simulink model "sensor_model"  (R2021a)
settings: Solver=FixedStepDiscrete  StartTime=0  StopTime=10.0  FixedStep=T_sample_control  RelTol=1e-3  EnableMultiTasking=on
model workspace (MAT data in the model file):
  CG = [0 0 0]
  g = [0 0 -9.81]
  t_sensor = 0.001
undefined symbols (not defined in the file or in its folder): DiscIntNeverNeededParam
libraries: rotations_lib x6, mspfiltlib x2, mspsensorlib x2, robotcorelib x2, aerolibcommonsys x1
settings Model: DataDictionary=pid.sldd  EnableAccessToBaseWorkspace=off  ModifiedByFormat=The MathWorks Inc.  Creator=The MathWorks, Inc.  LastModifiedBy=The MathWorks Inc.
settings SolverCC: ZeroCrossControl=DisableAll  AlgebraicLoopSolver=TrustRegion
settings DataIOCC: SaveFormat=StructureWithTime  SaveOutput=off  SaveTime=off  ReturnWorkspaceOutputs=off
settings OptimizationCC: BlockReduction=off  DefaultParameterBehavior=Inlined  InlineInvariantSignals=on  BufferReuse=off  PassReuseOutputArgsAs=Individual arguments  ExpressionDepthLimit=2147483647  ZeroExternalMemoryAtStartup=off  ZeroInternalMemoryAtStartup=off  EfficientFloat2IntCast=on  LifeSpan=1  EfficientTunableParamExpr=on
settings DebuggingCC: AlgebraicLoopMsg=none  FcnCallInpInsideContextMsg=warning  UnconnectedInputMsg=none  UnconnectedOutputMsg=none  UnconnectedLineMsg=none  UniqueDataStoreMsg=error  AssertControl=DisableAll  AllowSymbolicDim=off  StateNameClashWarn=warning  StrictBusMsg=ErrorOnBusTreatedAsVector  SFUnexpectedBacktrackingDiag=warning  SFNoUnconditionalDefaultTransitionDiag=warning  SFExecutionAtInitializationDiag=none  SFMachineParentedDataDiag=warning  ArithmeticOperatorsInVariantConditions=warning
settings HardwareCC: ProdBitPerPointer=32  ProdBitPerSizeT=32  ProdBitPerPtrDiffT=32  ProdLargestAtomicFloat=None  ProdIntDivRoundTo=Undefined  ProdEndianess=Unspecified  ProdWordSize=32  ProdHWDeviceType=32-bit Generic
settings ModelReferenceCC: PropagateSignalLabelsOutOfModel=off
settings SFSimCC: SimUseLocalCustomCode=off  CustomCodeUndefinedFunction=UseInterfaceOnly
settings RTWCC: SystemTargetFile=ert.tlc  TemplateMakefile=ert_default_tmf  GenerateReport=on  RTWUseLocalCustomCode=off  IncludeHyperlinkInReport=on  GenerateTraceInfo=on  GenerateTraceReport=on  GenerateTraceReportSl=on  GenerateTraceReportSf=on  GenerateTraceReportEml=on  GenerateCodeMetricsReport=on
settings CodeAppCC: IgnoreCustomStorageClasses=off  IgnoreTestpoints=on  CustomSymbolStrType=$N$R$M  StateflowObjectComments=on  InternalIdentifier=Classic
settings ERTTargetCC: MultiwordLength=2048  GenerateSampleERTMain=on  CombineOutputUpdateFcns=off  SupportNonFinite=off  ParenthesesLevel=Maximum  InlinedParameterPlacement=NonHierarchical  ERTCustomFileTemplate=example_file_process.tlc  ConvertIfToSwitch=off  SuppressUnreachableDefaultCases=off
settings ConfigComp: CovMetricSettings=dw  CovSaveCumulativeToWorkspaceVar=on  CovSaveSingleToWorkspaceVar=on  CovExternalEMLEnable=off  CovSFcnEnable=off

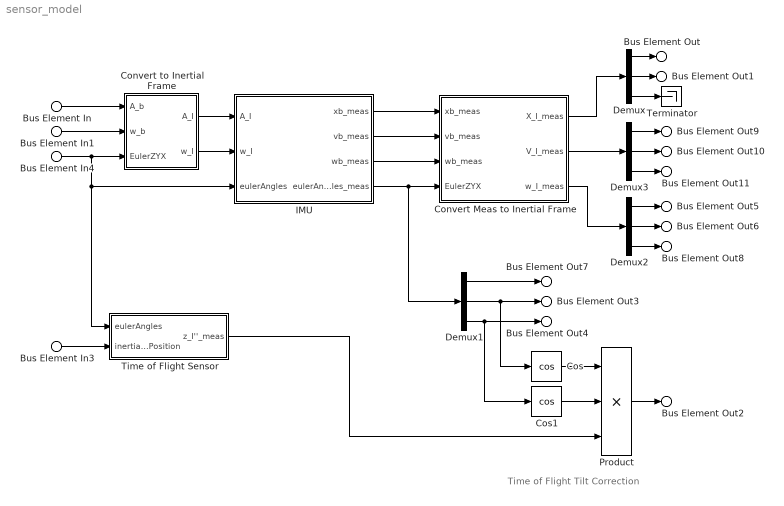
== system sensor_model ==
  note: Time of Flight Tilt Correction
  Bus Element In : Inport  PortName=6DOF  Element=body.acceleration
  Bus Element In1 : Inport  PortName=6DOF  Element=body.angularRate
  Bus Element In4 : Inport  PortName=6DOF  Element=body.angles
  Bus Element In3 : Inport  PortName=6DOF  Element=inertial.position
  Convert Meas to Inertial Frame : Subsystem
  Convert to Inertial Frame : Subsystem
  Cos : Trigonometry  Operator=cos
  Cos1 : Trigonometry  Operator=cos
  Demux{,1..3} (4 alike) : Demux  Outputs=3
  IMU : Subsystem  Description=Model approximating the SparkFun 9DoF IMU (ICM-20948) which will be used to determine the XY position and velocity and the attitude and angular rates of the flyer. The model uses the IMU and Attitude and Heading Reference System (AHRS) Simulink blocks to simulate our sensor.
  Product : Product  Inputs=3
  Terminator : Terminator
  Time of Flight Sensor : Subsystem  Description=A simulation model of the VL53L1X Time of Flight (ToF) sensor which determines the distance of the MFWF to the ground.
  Bus Element Out : Outport  PortName=sensor_meas  Element=x
  Bus Element Out1 : Outport  PortName=sensor_meas  Element=y
  Bus Element Out7 : Outport  PortName=sensor_meas  Element=psi
  Bus Element Out3 : Outport  PortName=sensor_meas  Element=theta
  Bus Element Out4 : Outport  PortName=sensor_meas  Element=phi
  Bus Element Out5 : Outport  PortName=sensor_meas  Element=p
  Bus Element Out6 : Outport  PortName=sensor_meas  Element=q
  Bus Element Out8 : Outport  PortName=sensor_meas  Element=r
  Bus Element Out9 : Outport  PortName=sensor_meas  Element=Vx
  Bus Element Out10 : Outport  PortName=sensor_meas  Element=Vy
  Bus Element Out11 : Outport  PortName=sensor_meas  Element=Vz
  Bus Element Out2 : Outport  PortName=sensor_meas  Element=z
  wires:
  Demux/1 -> Bus Element Out/1
  Demux3/3 -> Bus Element Out11/1
  Demux/3 -> Terminator/1
  Demux2/2 -> Bus Element Out6/1
  Demux2/1 -> Bus Element Out5/1
  Demux1/2 -> Bus Element Out3/1, Cos/1
  Demux3/1 -> Bus Element Out9/1
  IMU/4(eulerAngles_meas) -> Demux1/1, Convert Meas to Inertial Frame/4(EulerZYX)
  Demux3/2 -> Bus Element Out10/1
  Demux/2 -> Bus Element Out1/1
  Demux2/3 -> Bus Element Out8/1
  Bus Element In3/1 -> Time of Flight Sensor/2(inertialPosition)
  Bus Element In/1 -> Convert to Inertial Frame/1(A_b)
  Bus Element In1/1 -> Convert to Inertial Frame/2(w_b)
  Convert to Inertial Frame/2(w_I) -> IMU/2(w_I)
  IMU/1(xb_meas) -> Convert Meas to Inertial Frame/1(xb_meas)
  IMU/2(vb_meas) -> Convert Meas to Inertial Frame/2(vb_meas)
  IMU/3(wb_meas) -> Convert Meas to Inertial Frame/3(wb_meas)
  Convert Meas to Inertial Frame/1(X_I_meas) -> Demux/1
  Convert Meas to Inertial Frame/3(w_I_meas) -> Demux2/1
  Cos/1 -> Product/1
  Time of Flight Sensor/1(z_I''_meas) -> Product/3
  Cos1/1 -> Product/2
  Product/1 -> Bus Element Out2/1
  Convert to Inertial Frame/1(A_I) -> IMU/1(A_I)
  Bus Element In4/1 -> Time of Flight Sensor/1(eulerAngles), IMU/3(eulerAngles), Convert to Inertial Frame/3(EulerZYX)
  Convert Meas to Inertial Frame/2(V_I_meas) -> Demux3/1
  Demux1/1 -> Bus Element Out7/1
  Demux1/3 -> Cos1/1, Bus Element Out4/1

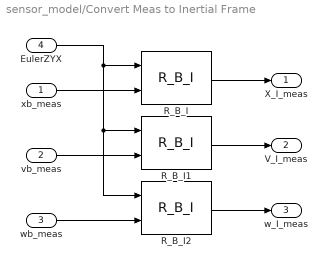
== system sensor_model/Convert Meas to Inertial Frame ==
  xb_meas : Inport
  vb_meas : Inport  Port=2
  wb_meas : Inport  Port=3
  EulerZYX : Inport  Port=4
  R_B_I : rotations_lib/R_B_I  SystemSampleTime=-1  VariantActivationTime=update diagram  Latency=0  AutoFrameSizeCalculation=off
  R_B_I1 : rotations_lib/R_B_I  SystemSampleTime=-1  VariantActivationTime=update diagram  Latency=0  AutoFrameSizeCalculation=off
  R_B_I2 : rotations_lib/R_B_I  SystemSampleTime=-1  VariantActivationTime=update diagram  Latency=0  AutoFrameSizeCalculation=off
  X_I_meas : Outport
  V_I_meas : Outport  Port=2
  w_I_meas : Outport  Port=3
  wires:
  EulerZYX/1 -> R_B_I2/1, R_B_I1/1, R_B_I/1
  xb_meas/1 -> R_B_I/2
  R_B_I/1 -> X_I_meas/1
  vb_meas/1 -> R_B_I1/2
  R_B_I1/1 -> V_I_meas/1
  R_B_I2/1 -> w_I_meas/1
  wb_meas/1 -> R_B_I2/2

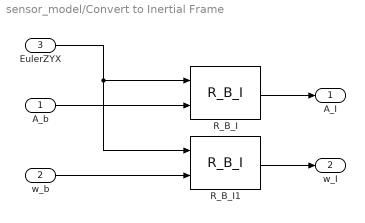
== system sensor_model/Convert to Inertial Frame ==
  A_b : Inport
  w_b : Inport  Port=2
  EulerZYX : Inport  Port=3
  R_B_I : rotations_lib/R_B_I  SystemSampleTime=-1  VariantActivationTime=update diagram  Latency=0  AutoFrameSizeCalculation=off
  R_B_I1 : rotations_lib/R_B_I  SystemSampleTime=-1  VariantActivationTime=update diagram  Latency=0  AutoFrameSizeCalculation=off
  A_I : Outport
  w_I : Outport  Port=2
  wires:
  EulerZYX/1 -> R_B_I1/1, R_B_I/1
  R_B_I/1 -> A_I/1
  A_b/1 -> R_B_I/2
  R_B_I1/1 -> w_I/1
  w_b/1 -> R_B_I1/2

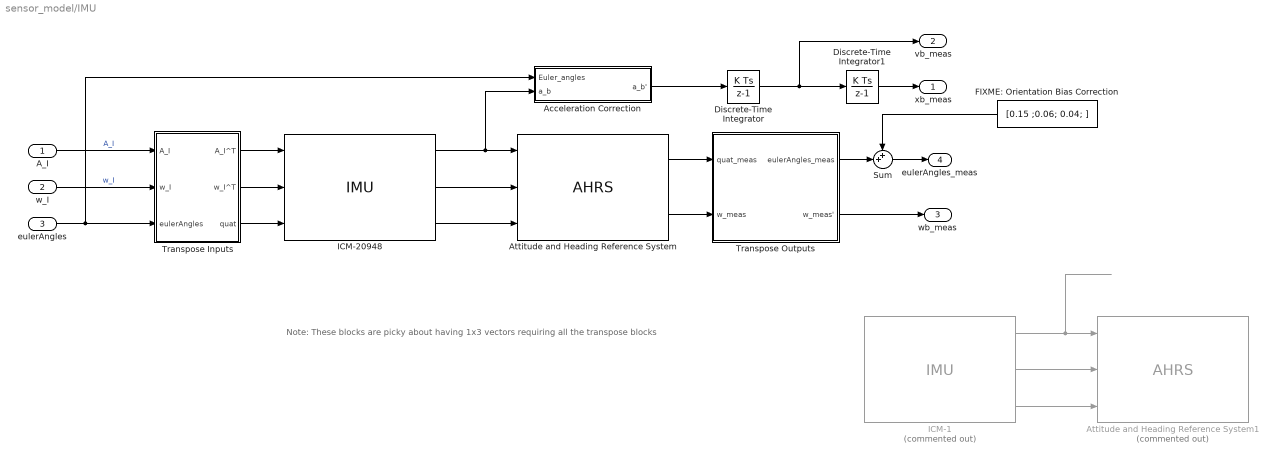
== system sensor_model/IMU ==
  note: Note: These blocks are picky about having 1x3 vectors requiring all the transpose blocks
  A_I : Inport
  w_I : Inport  Port=2
  eulerAngles : Inport  Port=3
  Acceleration Correction : Subsystem
  Attitude and Heading Reference System : mspfiltlib/AHRS  DispRefFrame=ENU  DecimationFactor=1  InitialProcessNoise=ahrsfilter.defaultProcessNoise  OrientationFormat=quaternion  SimulateUsing=Interpreted execution  AccelerometerNoise=0.0050625  GyroscopeNoise=6.84e-5  MagnetometerNoise=0.1e-15  GyroscopeDriftNoise=0.0872  LinearAccelerationNoise=0.55  MagneticDisturbanceNoise=0.3  LinearAccelerationDecayFactor=0.35  MagneticDisturbanceDecayFactor=0.3  ExpectedMagneticFieldStrength=50
      settings: SourceProductBaseCode=TF,NV
  Attitude and Heading Reference System1 : mspfiltlib/AHRS  Commented=on  DispRefFrame=ENU  DecimationFactor=1  InitialProcessNoise=ahrsfilter.defaultProcessNoise  OrientationFormat=quaternion  SimulateUsing=Interpreted execution  AccelerometerNoise=0.0050625  GyroscopeNoise=6.84e-5  MagnetometerNoise=0.1e-15  GyroscopeDriftNoise=0.0872  LinearAccelerationNoise=0.3  MagneticDisturbanceNoise=0.3  LinearAccelerationDecayFactor=0.3  MagneticDisturbanceDecayFactor=0.5  ExpectedMagneticFieldStrength=50
      settings: SourceProductBaseCode=TF,NV
  Discrete-Time Integrator : DiscreteIntegrator  SampleTime=-1  ICPrevOutput=DiscIntNeverNeededParam  ICPrevScaledInput=DiscIntNeverNeededParam
  Discrete-Time Integrator1 : DiscreteIntegrator  SampleTime=-1  ICPrevOutput=DiscIntNeverNeededParam  ICPrevScaledInput=DiscIntNeverNeededParam
  FIXME: Orientation Bias Correction : Constant  Value=[0.15 ;0.06; 0.04; ]
  ICM-1 : mspsensorlib/IMU  Commented=on  DispRefFrame=ENU  Temperature=25  MagneticFieldNED=[ 27.5550, -2.4169, -16.0849 ]  MagneticFieldENU=[ -2.4169, 27.5550, 16.0849 ]  SeedDouble=19  SimulateUsing=Interpreted execution  AccelParamsMeasurementRange=4*9.81  AccelParamsResolution=9.81/8192  AccelParamsConstantBias=[ 0, 0, 0 ]  AccelParamsAxesMisalignment=[ 0, 0, 0 ]  AccelParamsNoiseDensity=[ 230, 230, 230 ] * 9.81e-6  AccelParamsBiasInstability=[ 50, 50, 50] * 9.81e-3  AccelParamsRandomWalk=[ 230, 230, 230 ] * 9.81e-6  AccelParamsTemperatureBias=[ 0.8, 0.8, 0.8 ] * 9.81e-3  AccelParamsTemperatureScaleFactor=[0.026 0.026 0.026]  GyroParamsMeasurementRange=deg2rad(250)  GyroParamsResolution=1/deg2rad(131)  GyroParamsConstantBias=[ 0, 0, 0 ]  GyroParamsAxesMisalignment=[ 0, 0, 0 ]  GyroParamsAccelerationBias=[ 0, 0, 0 ]  GyroParamsNoiseDensity=[ deg2rad(0.015), deg2rad(0.015), deg2rad(0.015) ]  GyroParamsBiasInstability=[ deg2rad(5) , deg2rad(5), deg2rad(5) ]  GyroParamsRandomWalk=[ deg2rad(0.015), deg2rad(0.015), deg2rad(0.015) ]  GyroParamsTemperatureBias=[ deg2rad(0.05), deg2rad(0.05), deg2rad(0.05) ]  GyroParamsTemperatureScaleFactor=[ 3, 3, 3 ]  MagParamsMeasurementRange=4900  MagParamsResolution=0.15  MagParamsConstantBias=[ 0, 0, 0 ]  MagParamsAxesMisalignment=[ 0, 0, 0 ]  MagParamsNoiseDensity=[ 0, 0, 0 ]  MagParamsBiasInstability=[ 0, 0, 0 ]  MagParamsRandomWalk=[ 0, 0, 0 ]  MagParamsTemperatureBias=[ 0, 0, 0 ]  MagParamsTemperatureScaleFactor=[ 0, 0, 0 ]
      settings: SourceProductBaseCode=TF,NV
  ICM-20948 : mspsensorlib/IMU  DispRefFrame=ENU  Temperature=25  MagneticFieldNED=[ 27.5550, -2.4169, -16.0849 ]  MagneticFieldENU=[ -2.4169, 27.5550, 16.0849 ]  SeedDouble=19  SimulateUsing=Interpreted execution  AccelParamsMeasurementRange=4*9.81  AccelParamsResolution=9.81/8192  AccelParamsConstantBias=[ 0, 0, 0 ]  AccelParamsAxesMisalignment=[ 0, 0, 0 ]  AccelParamsNoiseDensity=[ 0, 0, 0 ] * 9.81e-6  AccelParamsBiasInstability=[ 0, 0, 0 ]* 9.81e-3  AccelParamsRandomWalk=[ 0, 0, 0 ]* 9.81e-6  AccelParamsTemperatureBias=[ 0, 0, 0 ]* 9.81e-3  AccelParamsTemperatureScaleFactor=[0.026 0.026 0.026]  GyroParamsMeasurementRange=deg2rad(250)  GyroParamsResolution=1/deg2rad(131)  GyroParamsConstantBias=[ 0, 0, 0 ]  GyroParamsAxesMisalignment=[ 0, 0, 0 ]  GyroParamsAccelerationBias=[ 0, 0, 0 ]  GyroParamsNoiseDensity=[ 0, 0, 0 ]  GyroParamsBiasInstability=[ 0, 0, 0 ]  GyroParamsRandomWalk=[ 0, 0, 0 ]  GyroParamsTemperatureBias=[ 0, 0, 0 ]  GyroParamsTemperatureScaleFactor=[ 0, 0, 0 ]  MagParamsMeasurementRange=4900  MagParamsResolution=0.15  MagParamsConstantBias=[ 0, 0, 0 ]  MagParamsAxesMisalignment=[ 0, 0, 0 ]  MagParamsNoiseDensity=[ 0, 0, 0 ]  MagParamsBiasInstability=[ 0, 0, 0 ]  MagParamsRandomWalk=[ 0, 0, 0 ]  MagParamsTemperatureBias=[ 0, 0, 0 ]  MagParamsTemperatureScaleFactor=[ 0, 0, 0 ]
      settings: SourceProductBaseCode=TF,NV
  Sum : Sum  Inputs=++|
  Transpose Inputs : Subsystem
  Transpose Outputs : Subsystem
  xb_meas : Outport
  vb_meas : Outport  Port=2
  wb_meas : Outport  Port=3
  eulerAngles_meas : Outport  Port=4
  wires:
  ICM-20948/1 -> Acceleration Correction/2(a_b), Attitude and Heading Reference System/1
  ICM-20948/2 -> Attitude and Heading Reference System/2
  ICM-20948/3 -> Attitude and Heading Reference System/3
  Discrete-Time Integrator1/1 -> xb_meas/1
  Discrete-Time Integrator/1 -> Discrete-Time Integrator1/1, vb_meas/1
  eulerAngles/1 -> Acceleration Correction/1(Euler_angles), Transpose Inputs/3(eulerAngles)
  A_I/1 -> Transpose Inputs/1(A_I)  "A_I"
  w_I/1 -> Transpose Inputs/2(w_I)  "w_I"
  Transpose Inputs/1(A_I^T) -> ICM-20948/1
  Transpose Inputs/2(w_I^T) -> ICM-20948/2
  Transpose Inputs/3(quat) -> ICM-20948/3
  Attitude and Heading Reference System/1 -> Transpose Outputs/1(quat_meas)
  Attitude and Heading Reference System/2 -> Transpose Outputs/2(w_meas)
  Transpose Outputs/1(eulerAngles_meas) -> Sum/2
  Transpose Outputs/2(w_meas') -> wb_meas/1
  FIXME: Orientation Bias Correction/1 -> Sum/1
  Acceleration Correction/1(a_b') -> Discrete-Time Integrator/1
  Sum/1 -> eulerAngles_meas/1
  ICM-1/3 -> Attitude and Heading Reference System1/3
  ICM-1/2 -> Attitude and Heading Reference System1/2
  ICM-1/1 -> Attitude and Heading Reference System1/1

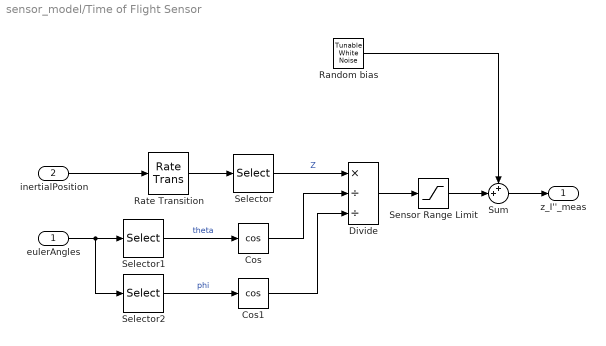
== system sensor_model/Time of Flight Sensor ==
  eulerAngles : Inport
  inertialPosition : Inport  Port=2
  Cos : Trigonometry  Operator=cos
  Cos1 : Trigonometry  Operator=cos
  Divide : Product  Inputs=*//
  Random bias : aerolibcommonsys/Tunable White Noise  pwr=0.0000001  Ts=t_sensor  seed=1337
      settings: SourceProductBaseCode=AE
  Rate Transition : RateTransition  OutPortSampleTime=t_sensor
  Selector : Selector  InputPortWidth=3  IndexOptions=Index vector (dialog)  Indices=[3]  OutputSizes=1
  Selector1 : Selector  InputPortWidth=3  IndexOptions=Index vector (dialog)  Indices=[2]  OutputSizes=1
  Selector2 : Selector  InputPortWidth=3  IndexOptions=Index vector (dialog)  Indices=[3]  OutputSizes=1
  Sensor Range Limit : Saturate  UpperLimit=2.2  LowerLimit=0
  Sum : Sum  Inputs=++|
  z_I''_meas : Outport
  wires:
  inertialPosition/1 -> Rate Transition/1
  Sum/1 -> z_I''_meas/1
  Selector/1 -> Divide/1  "Z"
  Random bias/1 -> Sum/1
  Rate Transition/1 -> Selector/1
  eulerAngles/1 -> Selector2/1, Selector1/1
  Selector1/1 -> Cos/1  "theta"
  Cos/1 -> Divide/2
  Divide/1 -> Sensor Range Limit/1
  Sensor Range Limit/1 -> Sum/2
  Selector2/1 -> Cos1/1  "phi"
  Cos1/1 -> Divide/3

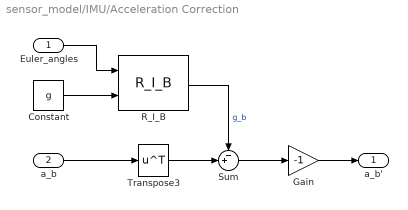
== system sensor_model/IMU/Acceleration Correction ==
  Euler_angles : Inport
  a_b : Inport  Port=2
  Constant : Constant  Value=g
  Gain : Gain  Gain=-1
  R_I_B : rotations_lib/R_I_B  SystemSampleTime=-1  VariantActivationTime=update diagram  Latency=0  AutoFrameSizeCalculation=off
  Sum : Sum  Inputs=-+|
  Transpose3 : Math  Operator=transpose  SaturateOnIntegerOverflow=on
  a_b' : Outport
  wires:
  Sum/1 -> Gain/1
  Transpose3/1 -> Sum/2
  a_b/1 -> Transpose3/1
  Gain/1 -> a_b'/1
  R_I_B/1 -> Sum/1  "g_b"
  Constant/1 -> R_I_B/2
  Euler_angles/1 -> R_I_B/1

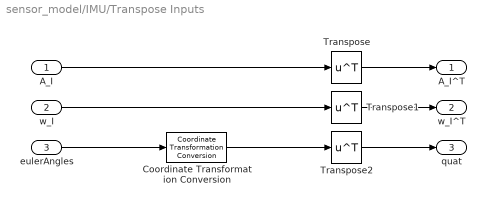
== system sensor_model/IMU/Transpose Inputs ==
  A_I : Inport
  w_I : Inport  Port=2
  eulerAngles : Inport  Port=3
  Coordinate Transformation Conversion : robotcorelib/Coordinate Transformation Conversion  InputRepresentation=Euler Angles  InputEulerSequence=ZYX  ShowTrVecInputPort=on  OutputRepresentation=Quaternion  OutputEulerSequence=ZYX  ShowTrVecOutputPort=on  SimulateUsing=Interpreted execution
      settings: SourceProductBaseCode=NV,RO,RR,UV
  Transpose : Math  Operator=transpose  SaturateOnIntegerOverflow=on
  Transpose1 : Math  Operator=transpose  SaturateOnIntegerOverflow=on
  Transpose2 : Math  Operator=transpose  SaturateOnIntegerOverflow=on
  A_I^T : Outport
  w_I^T : Outport  Port=2
  quat : Outport  Port=3
  wires:
  Transpose1/1 -> w_I^T/1
  Coordinate Transformation Conversion/1 -> Transpose2/1
  Transpose2/1 -> quat/1
  A_I/1 -> Transpose/1
  w_I/1 -> Transpose1/1
  eulerAngles/1 -> Coordinate Transformation Conversion/1
  Transpose/1 -> A_I^T/1

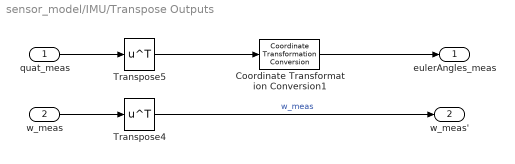
== system sensor_model/IMU/Transpose Outputs ==
  quat_meas : Inport
  w_meas : Inport  Port=2
  Coordinate Transformation Conversion1 : robotcorelib/Coordinate Transformation Conversion  InputRepresentation=Quaternion  InputEulerSequence=ZYX  ShowTrVecInputPort=on  OutputRepresentation=Euler Angles  OutputEulerSequence=ZYX  ShowTrVecOutputPort=on  SimulateUsing=Interpreted execution
      settings: SourceProductBaseCode=NV,RO,RR,UV
  Transpose4 : Math  Operator=transpose  SaturateOnIntegerOverflow=on
  Transpose5 : Math  Operator=transpose  SaturateOnIntegerOverflow=on
  eulerAngles_meas : Outport
  w_meas' : Outport  Port=2
  wires:
  Transpose5/1 -> Coordinate Transformation Conversion1/1
  Transpose4/1 -> w_meas'/1  "w_meas"
  quat_meas/1 -> Transpose5/1
  w_meas/1 -> Transpose4/1
  Coordinate Transformation Conversion1/1 -> eulerAngles_meas/1
